simulink model "Simu_Simulink"  (R2016a)
settings: Solver=FixedStepDiscrete  StartTime=0.0  StopTime=20  FixedStep=0.01  RelTol=1e-3
values from neighbouring files (symbols this model uses):
  lambdaSplit = reshape(lambda,lambdaDim,sizeSeg,DoP)    [Simu_Matlab.m]    (also in Simu_Simulink_Setup.m = reshape(lambda, lambdaDim,  sizeSeg,DoP))
  LAMBDASplit = reshape(LAMBDA,xDim,xDim,sizeSeg,DoP)    [Simu_Matlab.m]    (also in Simu_Simulink_Setup.m = reshape(LAMBDA, xDim, xDim, sizeSeg,DoP))
  muSplit = reshape(mu,muDim,sizeSeg,DoP)    [Simu_Matlab.m]    (also in Simu_Simulink_Setup.m = reshape(mu,     muDim,      sizeSeg,DoP))
  uSplit = reshape(u,uDim,sizeSeg,DoP)    [Simu_Matlab.m]    (also in Simu_Simulink_Setup.m = reshape(u,      uDim,       sizeSeg,DoP))
  x0 = [1 0]    [GEN_initData.mat]    (also in NMPC_Problem_Formulation.m = [1;0]; Simu_Matlab.m = SIM_Plant_RK4(uOpt(1,1),x0,pSimVal,Ts); Simu_Simulink_Setup.m = data.x0)
  xSplit = reshape(x,xDim,sizeSeg,DoP)    [Simu_Matlab.m]    (also in Simu_Simulink_Setup.m = reshape(x,      xDim,       sizeSeg,DoP))
settings Model: Creator=Deng  LastModifiedBy=Deng
settings OptimizationCC: SimCompilerOptimization=on
settings HardwareCC: ProdWordSize=32  ProdHWDeviceType=Specified
settings SFSimCC: SimCustomHeaderCode="#include \"NMPC_Iter.h\""  SimUserIncludeDirs=./codegen/dll/NMPC_Iter  SimUserLibraries=NMPC_Iter.lib
settings RTWCC: GenerateReport=on  RTWUseSimCustomCode=on  CustomHeaderCode="#include \"NMPC_Iter.h\""  CustomInclude=./codegen/dll/NMPC_Iter  CustomLibrary=NMPC_Iter.lib  BuildConfiguration=Faster Runs  LaunchReport=on

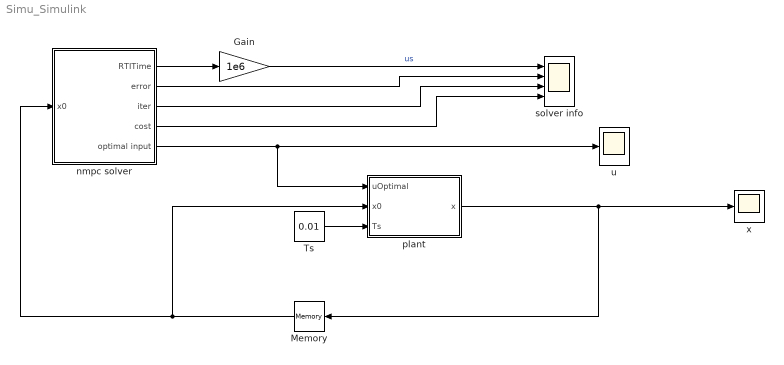
== system Simu_Simulink ==
  Gain : Gain  Gain=1e6
  Memory : Memory  X0=x0
  Ts : Constant  Value=0.01
  nmpc solver : Subsystem
  plant : MATLAB Function  TreatAsAtomicUnit=on
  solver info : Scope  NumInputPorts=4
  u : Scope
  x : Scope
  wires:
  Memory/1 -> nmpc solver/1(x0), plant/2(x0)
  plant/1(x) -> Memory/1, x/1
  Ts/1 -> plant/3(Ts)
  nmpc solver/5(optimal input) -> u/1, plant/1(uOptimal)
  nmpc solver/2(error) -> solver info/2
  nmpc solver/1(RTITime) -> Gain/1
  nmpc solver/4(cost) -> solver info/4
  nmpc solver/3(iter) -> solver info/3
  Gain/1 -> solver info/1  "us"

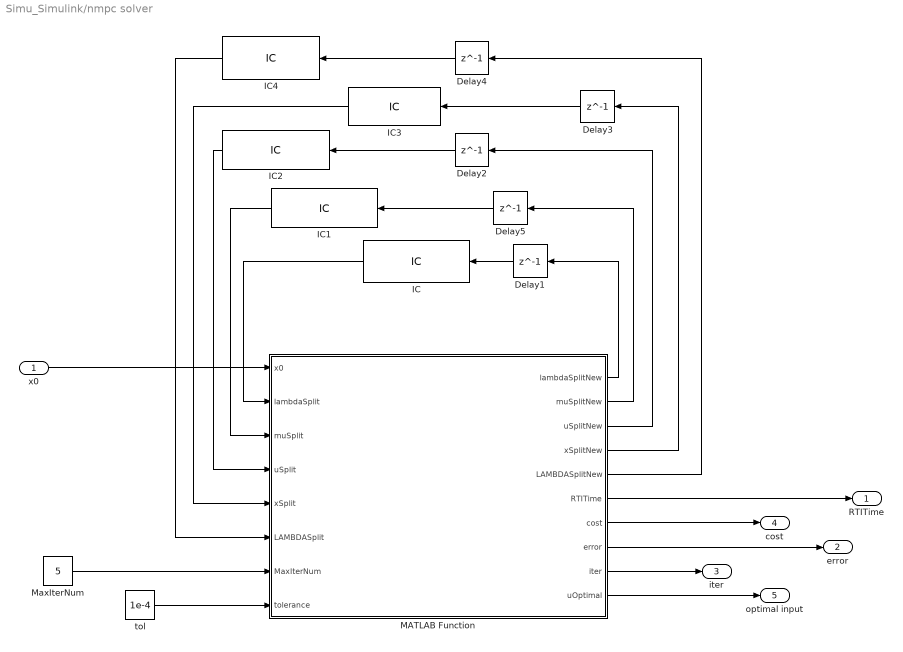
== system Simu_Simulink/nmpc solver ==
  x0 : Inport
  Delay{1..5} (5 alike) : Delay  DelayLength=1  InitialCondition=0
  IC : InitialCondition  Value=lambdaSplit
  IC1 : InitialCondition  Value=muSplit
  IC2 : InitialCondition  Value=uSplit
  IC3 : InitialCondition  Value=xSplit
  IC4 : InitialCondition  Value=LAMBDASplit
  MATLAB Function : MATLAB Function  TreatAsAtomicUnit=on
  MaxIterNum : Constant  Value=5
  tol : Constant  Value=1e-4
  RTITime : Outport
  error : Outport  Port=2
  iter : Outport  Port=3
  cost : Outport  Port=4
  optimal input : Outport  Port=5
  wires:
  Delay2/1 -> IC2/1
  Delay1/1 -> IC/1
  Delay4/1 -> IC4/1
  Delay3/1 -> IC3/1
  MaxIterNum/1 -> MATLAB Function/7(MaxIterNum)
  tol/1 -> MATLAB Function/8(tolerance)
  MATLAB Function/6(RTITime) -> RTITime/1
  MATLAB Function/7(cost) -> cost/1
  MATLAB Function/8(error) -> error/1
  MATLAB Function/10(uOptimal) -> optimal input/1
  x0/1 -> MATLAB Function/1(x0)
  MATLAB Function/9(iter) -> iter/1
  MATLAB Function/1(lambdaSplitNew) -> Delay1/1
  MATLAB Function/3(uSplitNew) -> Delay2/1
  MATLAB Function/4(xSplitNew) -> Delay3/1
  MATLAB Function/5(LAMBDASplitNew) -> Delay4/1
  IC/1 -> MATLAB Function/2(lambdaSplit)
  IC2/1 -> MATLAB Function/4(uSplit)
  IC3/1 -> MATLAB Function/5(xSplit)
  IC4/1 -> MATLAB Function/6(LAMBDASplit)
  Delay5/1 -> IC1/1
  IC1/1 -> MATLAB Function/3(muSplit)
  MATLAB Function/2(muSplitNew) -> Delay5/1

== matlab function Simu_Simulink/plant ==
  data: uOptimal input; x output; x0 input; Ts input
function x = plant(uOptimal,x0,Ts)
%#codegen
pSimVal = zeros(0,1);
x = SIM_Plant_RK4(uOptimal(1),x0,pSimVal,Ts);

== matlab function Simu_Simulink/nmpc solver/MATLAB Function ==
  data: lambdaSplitNew output; muSplitNew output; uSplitNew output; xSplitNew output; LAMBDASplitNew output; RTITime output; cost output; error output; iter output; uOptimal output; x0 input; lambdaSplit input; muSplit input; uSplit input; xSplit input; LAMBDASplit input; MaxIterNum input; tolerance input
function [lambdaSplitNew,muSplitNew,uSplitNew, xSplitNew, LAMBDASplitNew,...
          RTITime, cost, error, iter, uOptimal] = ...
            nmpc_solver( x0,lambdaSplit,muSplit,uSplit,...
                         xSplit,...
                         LAMBDASplit,...
                         MaxIterNum,...
                         tolerance)
%#codegen
cost = 0;
error = 0;
timeElapsed = 0;
RTITime = 0;
coder.ceval('NMPC_Iter_initialize');
for iter=1:MaxIterNum
    % Executing in generated code, call C function 
    coder.ceval('NMPC_Iter',...
                 x0,...
                 coder.ref(lambdaSplit),...
                 coder.ref(muSplit),...
                 coder.ref(uSplit),...
                 coder.ref(xSplit),...
                 coder.ref(LAMBDASplit),...
                 coder.wref(cost),...
                 coder.wref(error),...
                 coder.wref(timeElapsed));
    RTITime = RTITime + timeElapsed;
    if error<tolerance
        break;
    end
end
coder.ceval('NMPC_Iter_terminate');
lambdaSplitNew = lambdaSplit;
muSplitNew = muSplit;
uSplitNew = uSplit;
xSplitNew = xSplit;
LAMBDASplitNew = LAMBDASplit;
uOptimal = uSplit(:,1,1);
